simulink subsystem "No_IMU_Sensor"  (R2025b)
settings: Solver=VariableStepAuto  StartTime=0.0  StopTime=10.0  RelTol=1e-3
settings Model: Creator=The MathWorks, Inc.  LastModifiedBy=The MathWorks, Inc.
settings RTWCC: GPUComputeCapability=3.5

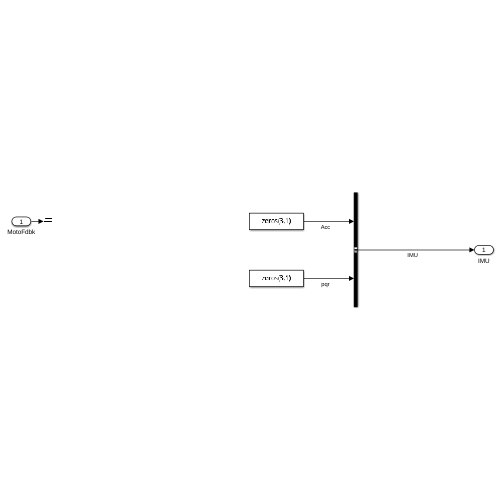
[thumbnail: Simulink's stored preview of the top-level diagram]
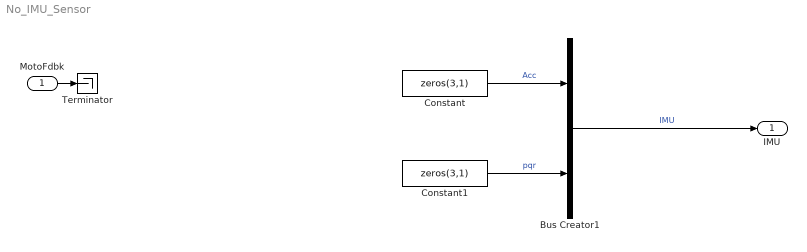
== system No_IMU_Sensor ==
  MotoFdbk : Inport
  Bus Creator1 : BusCreator  Inputs=2
  Constant : Constant  Value=zeros(3,1)  SampleTime=-1
  Constant1 : Constant  Value=zeros(3,1)  SampleTime=-1
  Terminator : Terminator
  IMU : Outport
  wires:
  Constant/1 -> Bus Creator1/1  "Acc"
  Bus Creator1/1 -> IMU/1  "IMU"
  Constant1/1 -> Bus Creator1/2  "pqr"
  MotoFdbk/1 -> Terminator/1
